simulink model "obserwator_regulator_odstanu_mierzone"  (R2023a)
settings: Solver=VariableStepAuto  StartTime=0.0  StopTime=10.0  RelTol=1e-3
values from neighbouring files (symbols this model uses):
  K = acker(A, B, [sb, sb, sb])    [do_workspace.m]    (also in zadania_1_5.m)
  L = acker(A', C', [s0, s0, s0])    [do_workspace.m]    (also in zadania_1_5.m)
settings Model: Creator=adams  LastModifiedBy=adams

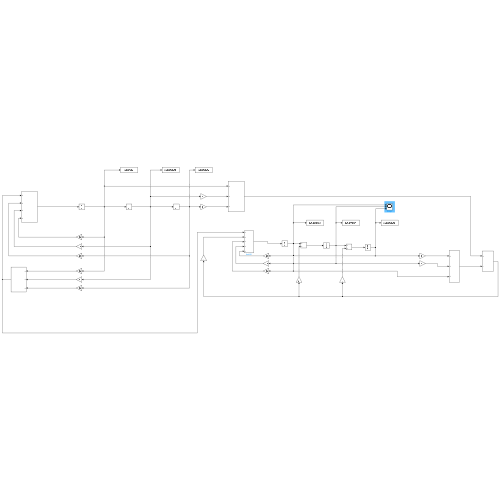
[thumbnail: Simulink's stored preview of the top-level diagram]
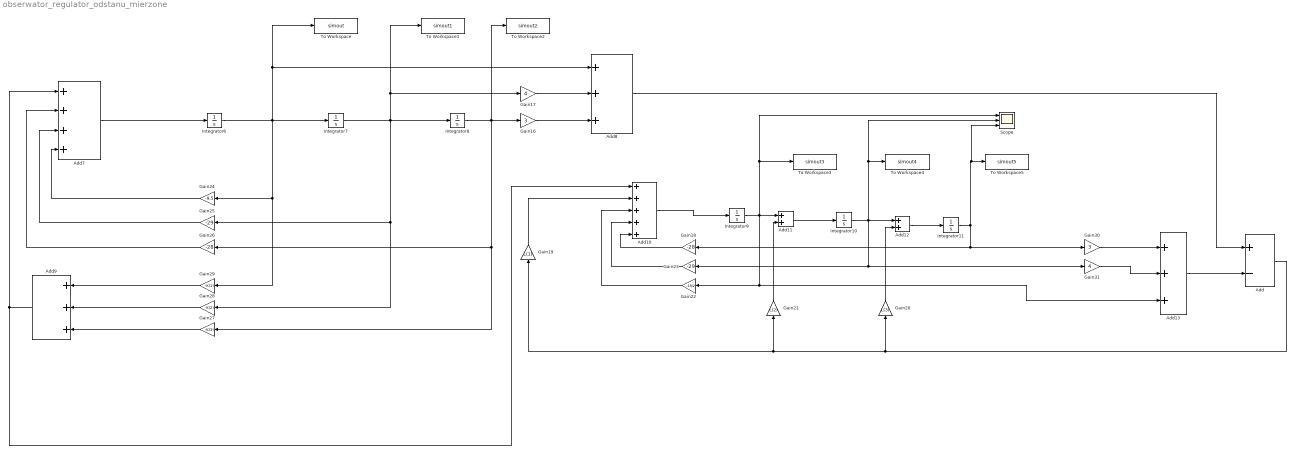
== system obserwator_regulator_odstanu_mierzone ==
  Add : Sum  Inputs=+-
  Add10 : Sum  Inputs=+++++
  Add11 : Sum
  Add12 : Sum
  Add13 : Sum  Inputs=+++
  Add7 : Sum  Inputs=++++
  Add8 : Sum  Inputs=+++
  Add9 : Sum  Inputs=+++
  Gain16 : Gain  Gain=3
  Gain17 : Gain  Gain=4
  Gain18 : Gain  Gain=-28
  Gain19 : Gain  Gain=L(1)
  Gain20 : Gain  Gain=L(3)
  Gain21 : Gain  Gain=L(2)
  Gain22 : Gain  Gain=-19/2
  Gain23 : Gain  Gain=-29
  Gain24 : Gain  Gain=-9.5
  Gain25 : Gain  Gain=-29
  Gain26 : Gain  Gain=-28
  Gain27 : Gain  Gain=-K(3)
  Gain28 : Gain  Gain=-K(2)
  Gain29 : Gain  Gain=-K(1)
  Gain30 : Gain  Gain=3
  Gain31 : Gain  Gain=4
  Integrator10 : Integrator  InitialCondition=20
  Integrator11 : Integrator  InitialCondition=30
  Integrator6 : Integrator  InitialCondition=-1
  Integrator7 : Integrator  InitialCondition=-1
  Integrator8 : Integrator  InitialCondition=2
  Integrator9 : Integrator  InitialCondition=10
  Scope : Scope  NumInputPorts=3
  To Workspace : ToWorkspace  VariableName=simout  SaveFormat=Structure With Time  SampleTime=-1
  To Workspace1 : ToWorkspace  VariableName=simout1  SaveFormat=Structure With Time  SampleTime=-1
  To Workspace2 : ToWorkspace  VariableName=simout2  SaveFormat=Structure With Time  SampleTime=-1
  To Workspace3 : ToWorkspace  VariableName=simout3  SaveFormat=Structure With Time  SampleTime=-1
  To Workspace4 : ToWorkspace  VariableName=simout4  SaveFormat=Structure With Time  SampleTime=-1
  To Workspace5 : ToWorkspace  VariableName=simout5  SaveFormat=Structure With Time  SampleTime=-1
  wires:
  Gain19/1 -> Add10/2
  Add7/1 -> Integrator6/1
  Gain28/1 -> Add9/2
  Integrator11/1 -> Scope/3, To Workspace5/1, Gain30/1, Gain18/1
  Integrator8/1 -> To Workspace2/1, Gain27/1, Gain26/1, Gain16/1
  Gain18/1 -> Add10/5
  Add9/1 -> Add7/1, Add10/1
  Gain29/1 -> Add9/1
  Integrator6/1 -> Gain29/1, Gain24/1, To Workspace/1, Add8/1, Integrator7/1
  Gain27/1 -> Add9/3
  Gain21/1 -> Add11/2
  Gain25/1 -> Add7/3
  Integrator7/1 -> Integrator8/1, Gain28/1, Gain25/1, To Workspace1/1, Gain17/1
  Gain24/1 -> Add7/4
  Gain16/1 -> Add8/3
  Add12/1 -> Integrator11/1
  Gain20/1 -> Add12/2
  Add11/1 -> Integrator10/1
  Add10/1 -> Integrator9/1
  Integrator9/1 -> Scope/1, To Workspace3/1, Add13/3, Gain22/1, Add11/1
  Gain22/1 -> Add10/3
  Integrator10/1 -> Scope/2, To Workspace4/1, Gain23/1, Gain31/1, Add12/1
  Gain23/1 -> Add10/4
  Gain26/1 -> Add7/2
  Gain17/1 -> Add8/2
  Gain31/1 -> Add13/2
  Gain30/1 -> Add13/1
  Add13/1 -> Add/2
  Add8/1 -> Add/1
  Add/1 -> Gain20/1, Gain21/1, Gain19/1
